simulink model "gmp_pmsm_sensored_nonlinear_sil_mdl_2022b"  (R2022b)
settings: Solver=VariableStepAuto  StartTime=0.0  StopTime=10  RelTol=1e-3
model workspace (MAT data in the model file):
  B = 0
  BW_i = 800
  Flux_t = 0.05895
  IQ24 : Simulink.NumericType (value not decoded)
  J = 0.018
  K_d = 3.72061852168
  K_m = 0.128242020589
  K_u = 0.00236407598332
  Ki_id = 0.001
  Ki_iq = 1
  Ki_n = 25225.1136556
  Kp_id = 1e-05
  Kp_iq = 5e-05
  Kp_n = 12.6125568278
  Ld_t = 0.00303
  Lq_t = 0.02019
  Max_p = 0.006000830667
  P = 2
  RLS_ini_a = 1000000
  Rd_mos = 0.01
  Rs = 0.1215
  Rv = 6.4
  T_final = 0
  T_initial = 0
  Tes = [4 7 10 7 4]
  Tf_t = 0.1
  Tm = 0
  Udq_limit = 550
  Var = 0
  Vce0 = 0
  Vd0 = 0
  Vdc = 80
  button = 1
  im_limit = 40
  mean_prd = 10
  position_init = 0.2
  r_ce = 1e-08
  r_d = 1e-08
  sample_prd = 100
  step_time = 0.2
  ts = 6.25e-05
  wc = 3500
libraries: peripheral_utilities x12, spsSeriesRLCBranchLib x6, spsVoltageMeasurementLib x2, gmp_sil_core_pack x1, spsPermanentMagnetSynchronousMachineLib x1, spsdq0toabcLib x1, spsFourierLib x1, spsControlledVoltageSourceLib x1, spspowerguiLib x1
(part 2 of 2)

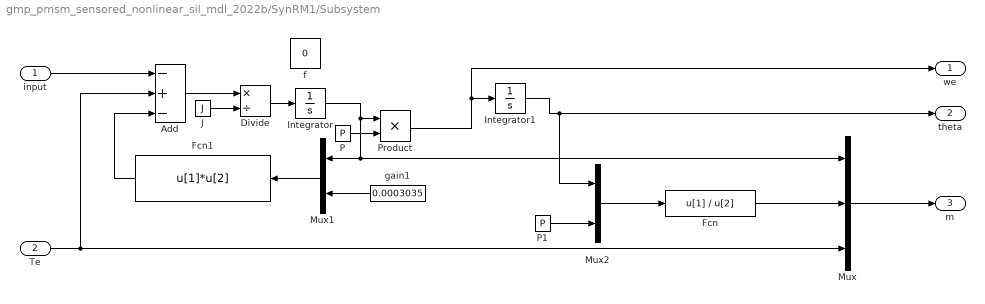
== system gmp_pmsm_sensored_nonlinear_sil_mdl_2022b/SynRM1/Subsystem ==
  input : Inport
  Te : Inport  Port=2
  Add : Sum  Inputs=-+-
  Divide : Product  Inputs=*/
  Fcn : Fcn  Expr=u[1] / u[2]
  Fcn1 : Fcn  Expr=u[1]*u[2]
  Integrator : Integrator
  Integrator1 : Integrator  InitialCondition=position_init
  J : Constant  Value=J  VectorParams1D=off
  Mux : Mux  Inputs=3
  Mux1 : Mux  Inputs=2
  Mux2 : Mux  Inputs=2
  P : Constant  Value=P
  P1 : Constant  Value=P
  Product : Product
  f : Constant  Value=0
  gain1 : Constant  Value=0.0003035
  we : Outport  VectorParamsAs1DForOutWhenUnconnected=off
  theta : Outport  Port=2  VectorParamsAs1DForOutWhenUnconnected=off
  m : Outport  Port=3  VectorParamsAs1DForOutWhenUnconnected=off
  wires:
  input/1 -> Add/1
  Te/1 -> Mux/3, Add/2
  J/1 -> Divide/2
  Add/1 -> Divide/1
  Divide/1 -> Integrator/1
  P/1 -> Product/2
  Integrator/1 -> Mux/1, Mux1/1, Product/1
  Integrator1/1 -> Mux2/1, theta/1
  Mux/1 -> m/1
  Mux1/1 -> Fcn1/1
  Fcn1/1 -> Add/3
  Mux2/1 -> Fcn/1
  Fcn/1 -> Mux/2
  P1/1 -> Mux2/2
  gain1/1 -> Mux1/2
  Product/1 -> we/1, Integrator1/1

== system gmp_pmsm_sensored_nonlinear_sil_mdl_2022b/SynRM1/Subsystem1 ==
  m_e : Inport
  m_m : Inport  Port=2
  Bus Creator : BusCreator  Inputs=13
  Demux : Demux  Outputs=[1, 1, 1]
  Demux1 : Demux  Outputs=[1, 1, 1, 1, 1, 1, 1, 1, 1, 1]
  Out : Outport  VectorParamsAs1DForOutWhenUnconnected=off
  wires:
  Demux1/1 -> Bus Creator/1  "Stator current is_a (A)"
  Demux1/2 -> Bus Creator/2  "Stator current is_b (A)"
  Demux1/3 -> Bus Creator/3  "Stator current is_c (A)"
  Demux1/4 -> Bus Creator/4  "Stator current is_q (A)"
  Demux1/5 -> Bus Creator/5  "Stator current is_d (A)"
  Demux1/6 -> Bus Creator/6  "Stator voltage Vs_q (V)"
  Demux1/7 -> Bus Creator/7  "Stator voltage Vs_d (V)"
  Demux1/8 -> Bus Creator/8  "Hall effect signal h_a"
  Demux1/9 -> Bus Creator/9  "Hall effect signal h_b"
  Demux1/10 -> Bus Creator/10  "Hall effect signal h_c"
  Demux/1 -> Bus Creator/11  "Rotor speed wm (rad/s)"
  Demux/2 -> Bus Creator/12  "Rotor angle thetam (rad)"
  Demux/3 -> Bus Creator/13  "Electromagnetic torque Te (N*m)"
  Bus Creator/1 -> Out/1
  m_m/1 -> Demux/1
  m_e/1 -> Demux1/1

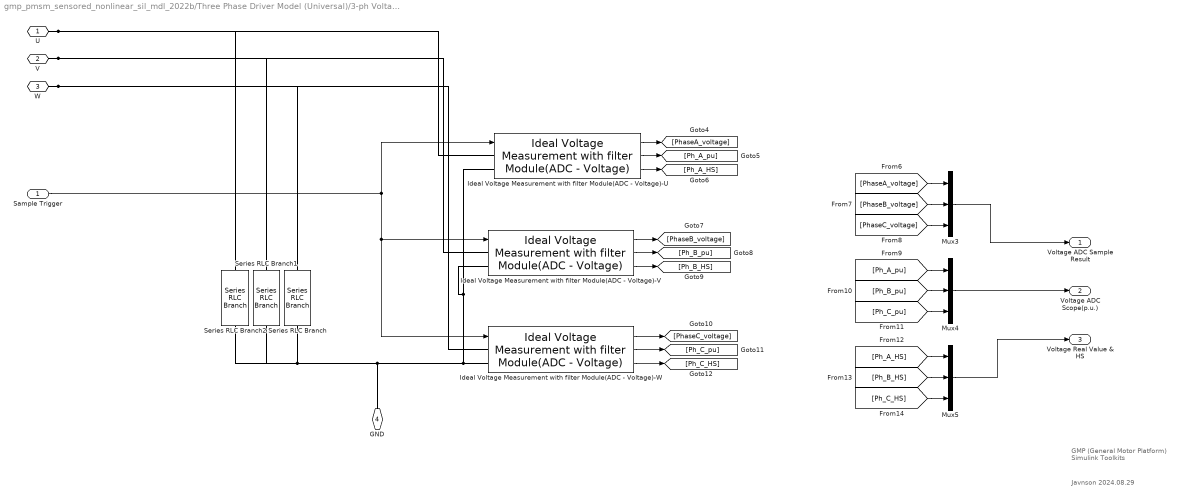
== system gmp_pmsm_sensored_nonlinear_sil_mdl_2022b/Three Phase Driver Model (Universal)/3-ph Voltage measurement ==
  note: Javnson
      | 2024.08.29
  note: GMP (General Motor Platform)
      | Simulink Toolkits
  Sample Trigger : Inport
  Ideal Voltage Measurement with filter Module(ADC - Voltage)-U : peripheral_utilities/Ideal Voltage Measurement with filter Module(ADC - Voltage)  ADC_GAIN=ADC_GAIN  ADC_BIT=ADC_BIT  ADC_REFERENCE=ADC_REFERENCE  ADC_BIAS=ADC_BIAS  ADC_INIT=ADC_INIT  cut_frequency=cut_frequency
      settings: SourceProductName=GMP Utilities Library
  Ideal Voltage Measurement with filter Module(ADC - Voltage)-V : peripheral_utilities/Ideal Voltage Measurement with filter Module(ADC - Voltage)  ADC_GAIN=ADC_GAIN  ADC_BIT=ADC_BIT  ADC_REFERENCE=ADC_REFERENCE  ADC_BIAS=ADC_BIAS  ADC_INIT=ADC_INIT  cut_frequency=cut_frequency
      settings: SourceProductName=GMP Utilities Library
  Ideal Voltage Measurement with filter Module(ADC - Voltage)-W : peripheral_utilities/Ideal Voltage Measurement with filter Module(ADC - Voltage)  ADC_GAIN=ADC_GAIN  ADC_BIT=ADC_BIT  ADC_REFERENCE=ADC_REFERENCE  ADC_BIAS=ADC_BIAS  ADC_INIT=ADC_INIT  cut_frequency=cut_frequency
      settings: SourceProductName=GMP Utilities Library
  Mux3 : Mux  Inputs=3
  Mux4 : Mux  Inputs=3
  Mux5 : Mux  Inputs=3
  Series RLC Branch : spsSeriesRLCBranchLib/Series RLC Branch  LConnTagsString=__new0  RConnTagsString=__new0  BranchType=R  Resistance=1e6  Inductance=1e-3  SetiL0=off  InitialCurrent=0  Capacitance=1e-6  Setx0=off  InitialVoltage=0  Measurements=None
  Series RLC Branch1 : spsSeriesRLCBranchLib/Series RLC Branch  LConnTagsString=__new0  RConnTagsString=__new0  BranchType=R  Resistance=1e6  Inductance=1e-3  SetiL0=off  InitialCurrent=0  Capacitance=1e-6  Setx0=off  InitialVoltage=0  Measurements=None
  Series RLC Branch2 : spsSeriesRLCBranchLib/Series RLC Branch  LConnTagsString=__new0  RConnTagsString=__new0  BranchType=R  Resistance=1e6  Inductance=1e-3  SetiL0=off  InitialCurrent=0  Capacitance=1e-6  Setx0=off  InitialVoltage=0  Measurements=None
  U : PMIOPort  Side=Left
  V : PMIOPort  Port=2  Side=Left
  W : PMIOPort  Port=3  Side=Left
  GND : PMIOPort  Port=4  Side=Left
  Voltage ADC Sample Result : Outport
  Voltage ADC Scope(p.u.) : Outport  Port=2
  Voltage Real Value & HS : Outport  Port=3
  wires:
  Ideal Voltage Measurement with filter Module(ADC - Voltage)-W/3 -> [Ph_C_HS]
  Sample Trigger/1 -> Ideal Voltage Measurement with filter Module(ADC - Voltage)-U/1, Ideal Voltage Measurement with filter Module(ADC - Voltage)-W/1, Ideal Voltage Measurement with filter Module(ADC - Voltage)-V/1
  Ideal Voltage Measurement with filter Module(ADC - Voltage)-V/2 -> [Ph_B_pu]
  Ideal Voltage Measurement with filter Module(ADC - Voltage)-V/3 -> [Ph_B_HS]
  Mux4/1 -> Voltage ADC Scope(p.u.)/1
  [Ph_B_HS] -> Mux5/2
  Ideal Voltage Measurement with filter Module(ADC - Voltage)-W/1 -> [PhaseC_voltage]
  Ideal Voltage Measurement with filter Module(ADC - Voltage)-V/1 -> [PhaseB_voltage]
  Ideal Voltage Measurement with filter Module(ADC - Voltage)-U/1 -> [PhaseA_voltage]
  Ideal Voltage Measurement with filter Module(ADC - Voltage)-U/2 -> [Ph_A_pu]
  [Ph_B_pu] -> Mux4/2
  [PhaseB_voltage] -> Mux3/2
  Ideal Voltage Measurement with filter Module(ADC - Voltage)-U/3 -> [Ph_A_HS]
  Ideal Voltage Measurement with filter Module(ADC - Voltage)-W/2 -> [Ph_C_pu]
  [Ph_A_pu] -> Mux4/1
  [PhaseC_voltage] -> Mux3/3
  [PhaseA_voltage] -> Mux3/1
  [Ph_C_pu] -> Mux4/3
  [Ph_C_HS] -> Mux5/3
  Mux3/1 -> Voltage ADC Sample Result/1
  [Ph_A_HS] -> Mux5/1
  Mux5/1 -> Voltage Real Value & HS/1
  connections:
  Ideal Voltage Measurement with filter Module(ADC - Voltage)-V/LConn2 -- Ideal Voltage Measurement with filter Module(ADC - Voltage)-U/LConn2 -- Series RLC Branch2/RConn1 -- Series RLC Branch1/RConn1 -- Series RLC Branch/RConn1 -- GND/RConn1 -- Ideal Voltage Measurement with filter Module(ADC - Voltage)-W/LConn2
  U/RConn1 -- Series RLC Branch2/LConn1 -- Ideal Voltage Measurement with filter Module(ADC - Voltage)-U/LConn1
  V/RConn1 -- Series RLC Branch1/LConn1 -- Ideal Voltage Measurement with filter Module(ADC - Voltage)-V/LConn1
  W/RConn1 -- Series RLC Branch/LConn1 -- Ideal Voltage Measurement with filter Module(ADC - Voltage)-W/LConn1

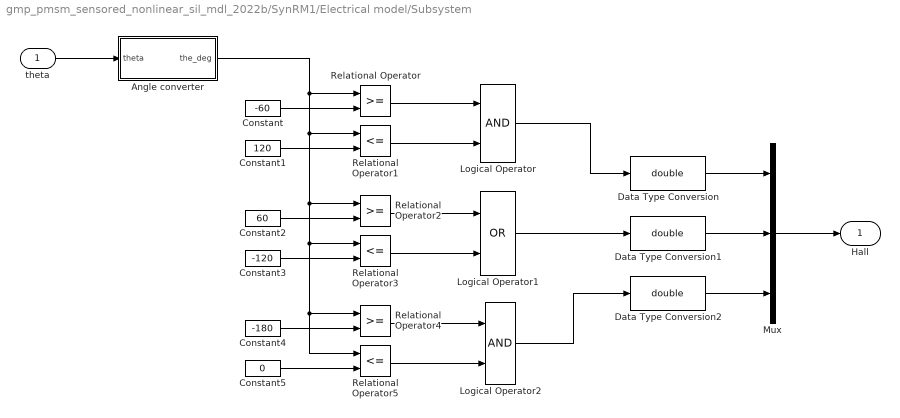
== system gmp_pmsm_sensored_nonlinear_sil_mdl_2022b/SynRM1/Electrical model/Subsystem ==
  theta : Inport
  Angle converter : Subsystem
  Constant : Constant  Value=-60
  Constant1 : Constant  Value=120
  Constant2 : Constant  Value=60
  Constant3 : Constant  Value=-120
  Constant4 : Constant  Value=-180
  Constant5 : Constant  Value=0
  Data Type Conversion : DataTypeConversion  OutDataTypeStr=double  SaturateOnIntegerOverflow=off
  Data Type Conversion1 : DataTypeConversion  OutDataTypeStr=double  SaturateOnIntegerOverflow=off
  Data Type Conversion2 : DataTypeConversion  OutDataTypeStr=double  SaturateOnIntegerOverflow=off
  Logical Operator : Logic  AllPortsSameDT=off  OutDataTypeStr=boolean
  Logical Operator1 : Logic  Operator=OR  AllPortsSameDT=off  OutDataTypeStr=boolean
  Logical Operator2 : Logic  AllPortsSameDT=off  OutDataTypeStr=boolean
  Mux : Mux  Inputs=3
  Relational Operator : RelationalOperator  OutDataTypeStr=boolean  RndMeth=Simplest  InputSameDT=off
  Relational Operator1 : RelationalOperator  Operator=<=  OutDataTypeStr=boolean  RndMeth=Simplest  InputSameDT=off
  Relational Operator2 : RelationalOperator  OutDataTypeStr=boolean  RndMeth=Simplest  InputSameDT=off
  Relational Operator3 : RelationalOperator  Operator=<=  OutDataTypeStr=boolean  RndMeth=Simplest  InputSameDT=off
  Relational Operator4 : RelationalOperator  OutDataTypeStr=boolean  RndMeth=Simplest  InputSameDT=off
  Relational Operator5 : RelationalOperator  Operator=<=  OutDataTypeStr=boolean  RndMeth=Simplest  InputSameDT=off
  Hall : Outport  VectorParamsAs1DForOutWhenUnconnected=off
  wires:
  theta/1 -> Angle converter/1(theta)
  Mux/1 -> Hall/1
  Data Type Conversion1/1 -> Mux/2
  Data Type Conversion/1 -> Mux/1
  Data Type Conversion2/1 -> Mux/3
  Logical Operator/1 -> Data Type Conversion/1
  Logical Operator2/1 -> Data Type Conversion2/1
  Logical Operator1/1 -> Data Type Conversion1/1
  Constant1/1 -> Relational Operator1/2
  Constant/1 -> Relational Operator/2
  Constant4/1 -> Relational Operator4/2
  Constant5/1 -> Relational Operator5/2
  Angle converter/1(the_deg) -> Relational Operator1/1, Relational Operator5/1, Relational Operator4/1, Relational Operator3/1, Relational Operator2/1, Relational Operator/1
  Constant2/1 -> Relational Operator2/2
  Constant3/1 -> Relational Operator3/2
  Relational Operator3/1 -> Logical Operator1/2
  Relational Operator2/1 -> Logical Operator1/1
  Relational Operator/1 -> Logical Operator/1
  Relational Operator1/1 -> Logical Operator/2
  Relational Operator4/1 -> Logical Operator2/1
  Relational Operator5/1 -> Logical Operator2/2

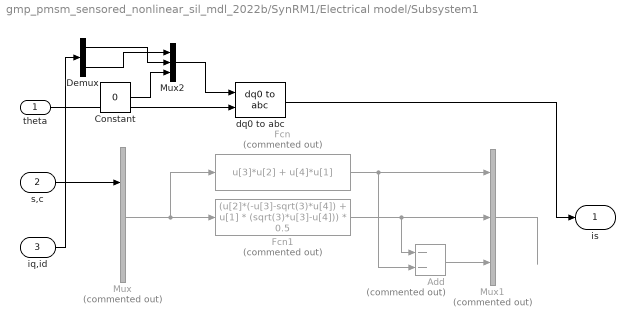
== system gmp_pmsm_sensored_nonlinear_sil_mdl_2022b/SynRM1/Electrical model/Subsystem1 ==
  theta : Inport
  s,c : Inport  Port=2
  iq,id : Inport  Port=3
  Add : Sum  Commented=on  Inputs=--
  Constant : Constant  Value=0
  Demux : Demux  Outputs=2
  Fcn : Fcn  Commented=on  Expr=u[3]*u[2] + u[4]*u[1]
  Fcn1 : Fcn  Commented=on  Expr=(u[2]*(-u[3]-sqrt(3)*u[4]) + u[1] * (sqrt(3)*u[3]-u[4])) * 0.5
  Mux : Mux  Commented=on  Inputs=[2, 2]
  Mux1 : Mux  Commented=on  Inputs=3
  Mux2 : Mux  Inputs=3
  dq0 to abc : spsdq0toabcLib/dq0 to abc  Alignment=Aligned with phase A axis
  is : Outport  VectorParamsAs1DForOutWhenUnconnected=off
  wires:
  s,c/1 -> Mux/1
  iq,id/1 -> Demux/1
  Fcn/1 -> Add/2, Mux1/1
  Fcn1/1 -> Add/1, Mux1/2
  Add/1 -> Mux1/3
  Mux/1 -> Fcn1/1, Fcn/1
  Mux1/1 -> ?
  theta/1 -> dq0 to abc/2
  Demux/1 -> Mux2/2
  Demux/2 -> Mux2/1
  Mux2/1 -> dq0 to abc/1
  dq0 to abc/1 -> is/1
  Constant/1 -> Mux2/3

== system gmp_pmsm_sensored_nonlinear_sil_mdl_2022b/SynRM1/Electrical model/Subsystem2 ==
  vq,vd : Inport
  we : Inport  Port=2
  LdLqRWb : Inport  Port=3
  Demux : Demux  Outputs=2
  Mux : Mux  Inputs=2
  Mux1 : Mux  Inputs=2
  id : Subsystem
  iq : Subsystem
  iq,id : Outport  VectorParamsAs1DForOutWhenUnconnected=off
  p_idiq_con : Outport  Port=2
  wires:
  Demux/1 -> iq/1(vq)
  id/1(id) -> iq/3(id), Mux/2
  we/1 -> iq/2(we), id/2(we)
  iq/1(iq) -> id/1(iq), Mux/1
  LdLqRWb/1 -> iq/4(LdLqRWb), id/4(LdLqRWb)
  Demux/2 -> id/3(vd)
  Mux/1 -> iq,id/1
  vq,vd/1 -> Demux/1
  iq/2(p_iq_con) -> Mux1/2
  id/2(p_id_con) -> Mux1/1
  Mux1/1 -> p_idiq_con/1

== system gmp_pmsm_sensored_nonlinear_sil_mdl_2022b/SynRM1/Electrical model/abc2qd ==
  "Vab, Vbc" : Inport
  theta : Inport  Port=2
  Mux : Mux  Inputs=2
  Mux1 : Mux  Inputs=[2, 2]
  Mux2 : Mux  Inputs=2
  Trigonometric Function : Trigonometry
  Trigonometric Function1 : Trigonometry  Operator=cos
  Vd : Fcn  Expr=( u[4]*(2*u[1]+u[2]) + (sqrt(3)*u[2]*u[3]) ) * 1/3
  Vq : Fcn  Expr=( -u[3]*(2*u[1]+u[2]) + (sqrt(3)*u[2]*u[4]) ) * 1/3
  "s, c" : Outport  VectorParamsAs1DForOutWhenUnconnected=off
  "vq, vd" : Outport  Port=2  VectorParamsAs1DForOutWhenUnconnected=off
  wires:
  Mux1/1 -> Vd/1, Vq/1
  Vd/1 -> Mux2/2
  Vq/1 -> Mux2/1
  Trigonometric Function/1 -> Mux/1
  Mux2/1 -> "vq, vd"/1
  Mux/1 -> "s, c"/1, Mux1/2
  theta/1 -> Trigonometric Function1/1, Trigonometric Function/1
  Trigonometric Function1/1 -> Mux/2
  "Vab, Vbc"/1 -> Mux1/1

== system gmp_pmsm_sensored_nonlinear_sil_mdl_2022b/SynRM1/Electrical model/Subsystem/Angle converter ==
  theta : Inport
  Gain : Gain  Gain=180/pi
  Trigonometric Function : Trigonometry
  Trigonometric Function1 : Trigonometry  Operator=cos
  Trigonometric Function2 : Trigonometry  Operator=atan2
  the_deg : Outport  VectorParamsAs1DForOutWhenUnconnected=off
  wires:
  Trigonometric Function1/1 -> Trigonometric Function2/2
  Gain/1 -> the_deg/1
  Trigonometric Function2/1 -> Gain/1
  Trigonometric Function/1 -> Trigonometric Function2/1
  theta/1 -> Trigonometric Function1/1, Trigonometric Function/1

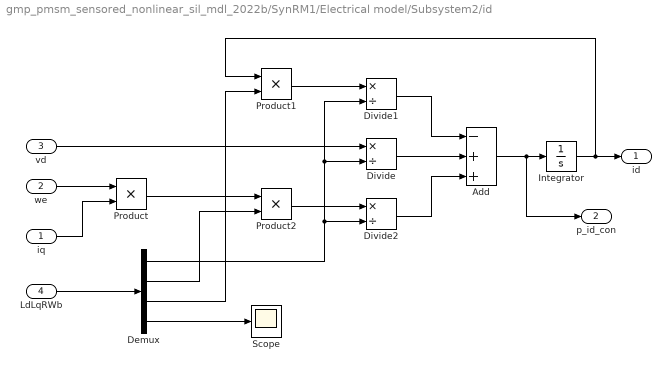
== system gmp_pmsm_sensored_nonlinear_sil_mdl_2022b/SynRM1/Electrical model/Subsystem2/id ==
  iq : Inport
  we : Inport  Port=2
  vd : Inport  Port=3
  LdLqRWb : Inport  Port=4
  Add : Sum  Inputs=-++
  Demux : Demux
  Divide : Product  Inputs=*/
  Divide1 : Product  Inputs=*/
  Divide2 : Product  Inputs=*/
  Integrator : Integrator
  Product : Product
  Product1 : Product
  Product2 : Product
  Scope : Scope
  id : Outport  VectorParamsAs1DForOutWhenUnconnected=off
  p_id_con : Outport  Port=2
  wires:
  we/1 -> Product/1
  iq/1 -> Product/2
  LdLqRWb/1 -> Demux/1
  Product/1 -> Product2/1
  Demux/2 -> Product2/2
  Demux/1 -> Divide1/2, Divide/2, Divide2/2
  Product2/1 -> Divide2/1
  vd/1 -> Divide/1
  Demux/3 -> Product1/2
  Integrator/1 -> Product1/1, id/1
  Add/1 -> p_id_con/1, Integrator/1
  Product1/1 -> Divide1/1
  Divide1/1 -> Add/1
  Divide/1 -> Add/2
  Divide2/1 -> Add/3
  Demux/4 -> Scope/1

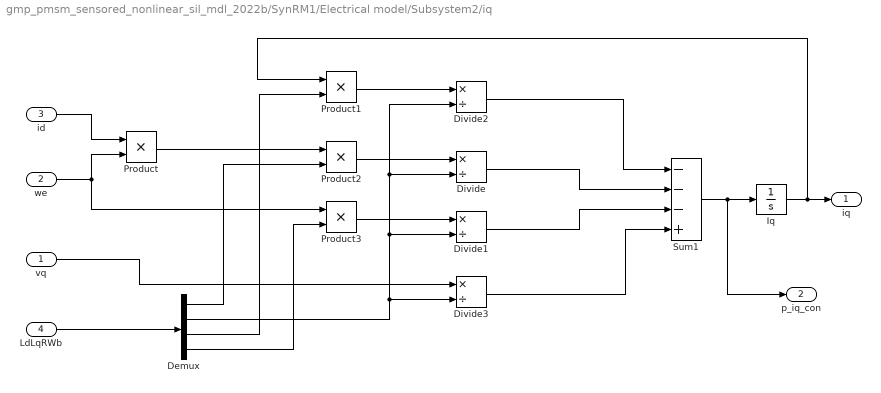
== system gmp_pmsm_sensored_nonlinear_sil_mdl_2022b/SynRM1/Electrical model/Subsystem2/iq ==
  vq : Inport
  we : Inport  Port=2
  id : Inport  Port=3
  LdLqRWb : Inport  Port=4
  Demux : Demux
  Divide{,1..3} (4 alike) : Product  Inputs=*/
  Iq : Integrator
  Product{,1..3} (4 alike) : Product
  Sum1 : Sum  Inputs=---+
  iq : Outport  VectorParamsAs1DForOutWhenUnconnected=off
  p_iq_con : Outport  Port=2
  wires:
  LdLqRWb/1 -> Demux/1
  Sum1/1 -> p_iq_con/1, Iq/1
  Iq/1 -> Product1/1, iq/1
  we/1 -> Product3/1, Product/2
  id/1 -> Product/1
  Demux/2 -> Divide1/2, Divide2/2, Divide/2, Divide3/2
  Product1/1 -> Divide2/1
  Demux/3 -> Product1/2
  Demux/1 -> Product2/2
  Product/1 -> Product2/1
  Demux/4 -> Product3/2
  vq/1 -> Divide3/1
  Divide2/1 -> Sum1/1
  Divide/1 -> Sum1/2
  Product2/1 -> Divide/1
  Product3/1 -> Divide1/1
  Divide1/1 -> Sum1/3
  Divide3/1 -> Sum1/4
